simulink model "BALANCEAMENTO_MEDIA"  (Simulink 7.5)
settings: Solver=ode45  StartTime=0.0  StopTime=40000  RelTol=1e-2
libraries: powerlib x49, simulink x1
settings Model: Creator=André  LastModifiedBy=André
settings SolverCC: ZeroCrossAlgorithm=Adaptive

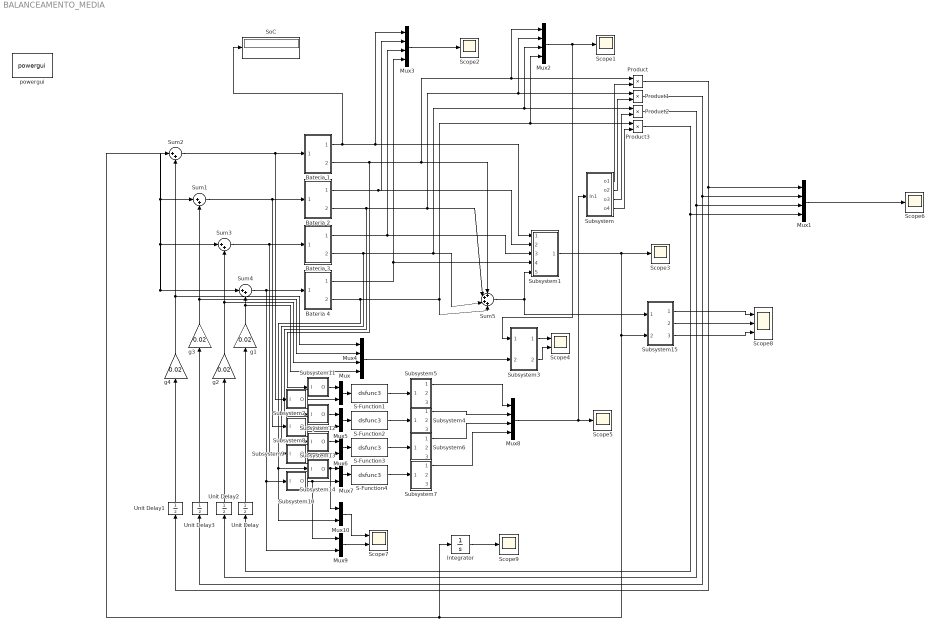
== system BALANCEAMENTO_MEDIA ==
  Bateria 1 : Subsystem
  Bateria 2 : Subsystem
  Bateria 3 : Subsystem
  Bateria 4 : Subsystem
  Integrator : Integrator
  Mux{,5..7,9..10} (6 alike) : Mux  Inputs=2
  Mux{1..4,8} (5 alike) : Mux
  Product{,1..3} (4 alike) : Product  OutDataType=fixdt(1, 16)  OutScaling=2^0  RndMeth=Zero
  S-Function{1..4} (4 alike) : S-Function  FunctionName=dsfunc3  Parameters="[0.5  0.01 0.01 1] %1 para UKF, 2 para EKF"  EnableBusSupport=off
  Scope{1..3,5..6,9} (6 alike) : Scope
      Scope1 settings: TimeRange=3600  YMin=3.34  YMax=3.361  SaveName=Volt
      Scope2 settings: TimeRange=1000  YMin=0.375  YMax=0.925  SaveName=SoC
      Scope3 settings: TimeRange=3600  YMin=0.40252  YMax=0.40262  SaveName=corrente
      Scope5 settings: TimeRange=1000  YMin=0.5  YMax=0.825  SaveName=SoC1
      Scope6 settings: TimeRange=3600  YMin=0  YMax=3.25  SaveName=ScopeData7
      Scope9 settings: TimeRange=1000  YMin=219  YMax=232  SaveName=CAP
  Scope4 : Scope  NumInputPorts=2
      settings: TimeRange=3600  YMin=0~7074.25  YMax=0.25~7076.75  SaveName=energia
  Scope7 : Scope  NumInputPorts=2
      settings: TimeRange=1000  YMin=3.025~0.325  YMax=3.225~0.5  SaveName=CV
  Scope8 : Scope  NumInputPorts=3
      settings: TimeRange=3600  YMin=-0.025~3350~-5  YMax=0.25~3800~5  SaveName=energia1
  SoC : Display
  Subsystem : Subsystem
  Subsystem1 : Subsystem
  Subsystem10 : Subsystem
  Subsystem11 : Subsystem
  Subsystem12 : Subsystem
  Subsystem13 : Subsystem
  Subsystem14 : Subsystem
  Subsystem15 : Subsystem
  Subsystem2 : Subsystem
  Subsystem3 : Subsystem
  Subsystem4 : Subsystem
  Subsystem5 : Subsystem
  Subsystem6 : Subsystem
  Subsystem7 : Subsystem
  Subsystem8 : Subsystem
  Subsystem9 : Subsystem
  Sum{1..4} (4 alike) : Sum  Inputs=|++  OutDataType=fixdt(1, 16)  OutScaling=2^0
  Sum5 : Sum  Inputs=++++  OutDataType=fixdt(1, 16)  OutScaling=2^0
  Unit Delay{,1..3} (4 alike) : UnitDelay  SampleTime=-1
  g{1..4} (4 alike) : Gain  Gain=0.02  ParameterDataType=fixdt(1, 16)  ParameterScaling=2^0  OutDataType=fixdt(1, 16)  OutScaling=2^0
  powergui : powerlib/powergui  Priority=1  SystemSampleTime=-1  SimulationMode=Continuous  SampleTime=50e-6  frequency=60  SPID=off  DisableSnubberDevices=off  DisableRonSwitches=off  DisableVfSwitches=off  SwTol=0  Interpol=off  frequencyindice=0  echomessages=off  HookPort=off  DisplayEquations=off  FunctionMessages=off  EnableUseOfTLC=off  x0status=blocks  RestoreLinks=warning  ResistiveCurrentMeasurement=off  Frange=[0:2:500]  Ylog=off  Xlog=on  ShowGrid=off  save=off  variable=ZData  ZoomFFT=on  StartTime=0.0  cycles=1  DisplayStyle=1  fundamental=60  FreqAxis=off  MaxFrequency=1000  frequencyindicesteady=1  RmsSteady=1  display=off  Ts=0  methode=off
  wires:
  Bateria 1/1(x _1) -> SoC/1, Mux3/1, Subsystem1/1(In1)
  Bateria 3/1(x _1) -> Mux3/3, Subsystem1/3(In3)
  Bateria 4/1(x _1) -> Mux3/4, Subsystem1/4(In4)
  Sum1/1 -> Bateria 2/1(u_1), Subsystem8/1(I)
  Subsystem/1(o1) -> Product/2
  Sum2/1 -> Bateria 1/1(u_1), Subsystem2/1(I)
  Subsystem/2(o2) -> Product1/2
  Sum3/1 -> Bateria 3/1(u_1), Subsystem9/1(I)
  Subsystem/3(o3) -> Product2/2
  Sum4/1 -> Bateria 4/1(u_1), Subsystem10/1(I), Mux9/2
  Subsystem/4(o4) -> Product3/2
  Bateria 1/2(y _1) -> Mux2/1, Product/1, Sum5/1, Subsystem11/1(I)
  Bateria 2/2(y _1) -> Product1/1, Mux2/2, Sum5/2, Subsystem12/1(I)
  Bateria 3/2(y _1) -> Product2/1, Mux2/3, Sum5/3, Subsystem13/1(I)
  Bateria 4/2(y _1) -> Product3/1, Mux2/4, Sum5/4, Subsystem14/1(I), Mux10/2
  Bateria 2/1(x _1) -> Mux3/2, Subsystem1/2(In2)
  Product3/1 -> Mux1/4, Unit Delay/1
  Product2/1 -> Mux1/3, Unit Delay2/1
  Product1/1 -> Mux1/2, Unit Delay3/1
  Product/1 -> Mux1/1, Unit Delay1/1
  g1/1 -> Sum4/2, Mux4/4
  g2/1 -> Sum3/2, Mux4/3
  g3/1 -> Sum1/2, Mux4/2
  g4/1 -> Sum2/2, Mux4/1
  Mux2/1 -> Scope1/1, Subsystem3/1(In1)
  Mux3/1 -> Scope2/1
  Sum5/1 -> Subsystem1/5(In5), Subsystem15/1(In1)
  Subsystem1/1(Corrente) -> Scope3/1, Subsystem15/2(In2), Sum2/1, Sum3/1, Sum4/1, Sum1/1, Integrator/1
  Mux1/1 -> Scope6/1
  Subsystem3/1(Pot) -> Scope4/1
  Subsystem3/2(Energ) -> Scope4/2
  Mux4/1 -> Subsystem3/2(In2)
  S-Function1/1 -> Subsystem5/1(1)
  Mux/1 -> S-Function1/1
  S-Function2/1 -> Subsystem4/1(1)
  Mux5/1 -> S-Function2/1
  S-Function3/1 -> Subsystem6/1(1)
  Mux6/1 -> S-Function3/1
  S-Function4/1 -> Subsystem7/1(1)
  Mux7/1 -> S-Function4/1
  Mux8/1 -> Scope5/1, Subsystem/1(In1)
  Subsystem5/1(1-) -> Mux8/1
  Subsystem4/1(1-) -> Mux8/2
  Subsystem6/1(1-) -> Mux8/3
  Subsystem7/1(1-) -> Mux8/4
  Unit Delay1/1 -> g4/1
  Unit Delay3/1 -> g3/1
  Unit Delay2/1 -> g2/1
  Unit Delay/1 -> g1/1
  Subsystem2/1(O) -> Mux/2
  Subsystem8/1(O) -> Mux5/2
  Subsystem9/1(O) -> Mux6/2
  Subsystem10/1(O) -> Mux7/2, Mux9/1
  Subsystem11/1(O) -> Mux/1
  Subsystem12/1(O) -> Mux5/1
  Subsystem13/1(O) -> Mux6/1
  Subsystem14/1(O) -> Mux7/1, Mux10/1
  Mux9/1 -> Scope7/2
  Mux10/1 -> Scope7/1
  Subsystem15/1(Pot) -> Scope8/1
  Subsystem15/2(Energ) -> Scope8/2
  Subsystem15/3(Energ1) -> Scope8/3
  Integrator/1 -> Scope9/1

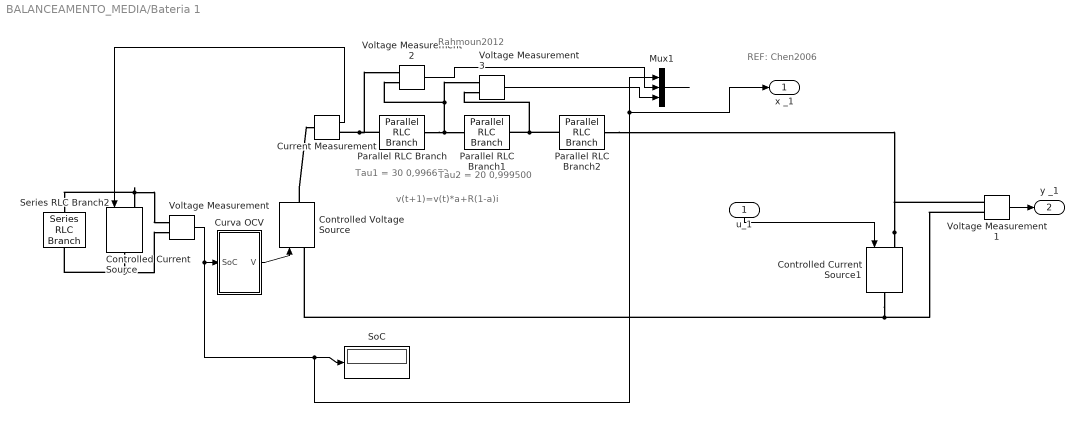
== system BALANCEAMENTO_MEDIA/Bateria 1 ==
  note: REF: Chen2006
  note: Tau1 = 30
      | 0,996672
  note: Tau2 = 20
      | 0,999500
  note: Rahmoun2012
  note: v(t+1)=v(t)*a+R(1-a)i
  u_1 : Inport
  Controlled Current Source : powerlib/Electrical Sources/Controlled Current Source  DialogController=POWERSYS.PowerSysDialog  SystemSampleTime=-1  Initialize=on  Source_Type=AC  Amplitude=0  Phase=0  Frequency=0  Measurements=None
  Controlled Current Source1 : powerlib/Electrical Sources/Controlled Current Source  DialogController=POWERSYS.PowerSysDialog  SystemSampleTime=-1  Initialize=on  Source_Type=DC  Amplitude=0  Phase=0  Frequency=0  Measurements=None
  Controlled Voltage Source : powerlib/Electrical Sources/Controlled Voltage Source  DialogController=POWERSYS.PowerSysDialog  SystemSampleTime=-1  Initialize=on  Source_Type=AC  Amplitude=0  Phase=0  Frequency=0  Measurements=None
  Current Measurement : powerlib/Measurements/Current Measurement  DialogController=POWERSYS.PowerSysDialog  SystemSampleTime=-1  PhasorSimulation=off  OutputType=Complex  PSBequivalent=0
  Curva OCV : Subsystem
  Mux1 : Mux  Inputs=3
  Parallel RLC Branch : powerlib/Elements/Parallel RLC Branch  DialogController=POWERSYS.PowerSysDialog  PhysicalDomain=powersysdomain  SubClassName=unknown  LeftPortType=p1  RightPortType=p1  LConnTagsString=a  RConnTagsString=__new0  BranchType=RC  Resistance=0.115  Inductance=1e-3  SetiL0=off  InitialCurrent=0  Capacitance=600  Setx0=off  InitialVoltage=0  Measurements=None
  Parallel RLC Branch1 : powerlib/Elements/Parallel RLC Branch  DialogController=POWERSYS.PowerSysDialog  PhysicalDomain=powersysdomain  SubClassName=unknown  LeftPortType=p1  RightPortType=p1  LConnTagsString=a  RConnTagsString=__new0  BranchType=RC  Resistance=0.066  Inductance=1e-3  SetiL0=off  InitialCurrent=0  Capacitance=409.1  Setx0=off  InitialVoltage=0  Measurements=None
  Parallel RLC Branch2 : powerlib/Elements/Parallel RLC Branch  DialogController=POWERSYS.PowerSysDialog  PhysicalDomain=powersysdomain  SubClassName=unknown  LeftPortType=p1  RightPortType=p1  LConnTagsString=a  RConnTagsString=__new0  BranchType=R  Resistance=0.174  Inductance=1e-3  SetiL0=off  InitialCurrent=0  Capacitance=1e-6  Setx0=off  InitialVoltage=0  Measurements=None
  Series RLC Branch2 : powerlib/Elements/Series RLC Branch  DialogController=POWERSYS.PowerSysDialog  PhysicalDomain=powersysdomain  SubClassName=unknown  LeftPortType=p1  RightPortType=p1  LConnTagsString=__new0  RConnTagsString=__new0  BranchType=C  Resistance=1  Inductance=1e-3  SetiL0=off  InitialCurrent=0  Capacitance=2070  Setx0=on  InitialVoltage=0.98  Measurements=None
  SoC : Display
  Voltage Measurement{,1..3} (4 alike) : powerlib/Measurements/Voltage Measurement  DialogController=POWERSYS.PowerSysDialog  SystemSampleTime=-1  PhasorSimulation=off  OutputType=Complex  PSBequivalent=0
  x _1 : Outport
  y _1 : Outport  Port=2
  wires:
  Voltage Measurement1/1 -> y _1/1
  Curva OCV/1(V) -> Controlled Voltage Source/1
  Voltage Measurement/1 -> Curva OCV/1(SoC), SoC/1, Mux1/1, x _1/1
  Current Measurement/1 -> Controlled Current Source/1
  u_1/1 -> Controlled Current Source1/1
  Mux1/1 -> ?
  Voltage Measurement2/1 -> Mux1/2
  Voltage Measurement3/1 -> Mux1/3
  connections:
  Controlled Current Source/LConn1 -- Voltage Measurement/LConn1 -- Series RLC Branch2/LConn1
  Controlled Current Source/RConn1 -- Voltage Measurement/LConn2 -- Series RLC Branch2/RConn1
  Controlled Current Source1/LConn1 -- Parallel RLC Branch2/RConn1 -- Voltage Measurement1/LConn1
  Controlled Current Source1/RConn1 -- Controlled Voltage Source/LConn1 -- Voltage Measurement1/LConn2
  Controlled Voltage Source/RConn1 -- Current Measurement/LConn1
  Parallel RLC Branch/LConn1 -- Current Measurement/RConn1 -- Voltage Measurement2/LConn1
  Parallel RLC Branch/RConn1 -- Parallel RLC Branch1/LConn1 -- Voltage Measurement2/LConn2 -- Voltage Measurement3/LConn1
  Parallel RLC Branch2/LConn1 -- Parallel RLC Branch1/RConn1 -- Voltage Measurement3/LConn2

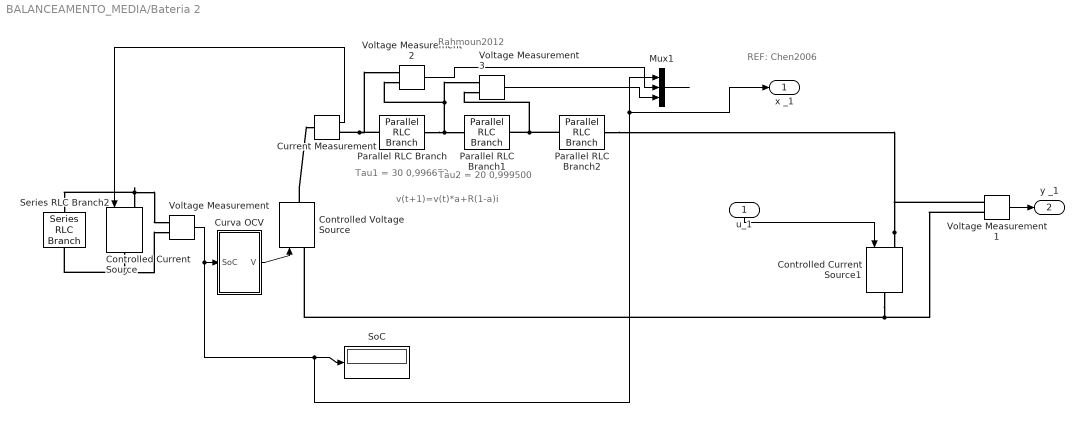
== system BALANCEAMENTO_MEDIA/Bateria 2 ==
  note: REF: Chen2006
  note: Tau1 = 30
      | 0,996672
  note: Tau2 = 20
      | 0,999500
  note: Rahmoun2012
  note: v(t+1)=v(t)*a+R(1-a)i
  u_1 : Inport
  Controlled Current Source : powerlib/Electrical Sources/Controlled Current Source  DialogController=POWERSYS.PowerSysDialog  SystemSampleTime=-1  Initialize=on  Source_Type=AC  Amplitude=0  Phase=0  Frequency=0  Measurements=None
  Controlled Current Source1 : powerlib/Electrical Sources/Controlled Current Source  DialogController=POWERSYS.PowerSysDialog  SystemSampleTime=-1  Initialize=on  Source_Type=DC  Amplitude=0  Phase=0  Frequency=0  Measurements=None
  Controlled Voltage Source : powerlib/Electrical Sources/Controlled Voltage Source  DialogController=POWERSYS.PowerSysDialog  SystemSampleTime=-1  Initialize=on  Source_Type=AC  Amplitude=0  Phase=0  Frequency=0  Measurements=None
  Current Measurement : powerlib/Measurements/Current Measurement  DialogController=POWERSYS.PowerSysDialog  SystemSampleTime=-1  PhasorSimulation=off  OutputType=Complex  PSBequivalent=0
  Curva OCV : Subsystem
  Mux1 : Mux  Inputs=3
  Parallel RLC Branch : powerlib/Elements/Parallel RLC Branch  DialogController=POWERSYS.PowerSysDialog  PhysicalDomain=powersysdomain  SubClassName=unknown  LeftPortType=p1  RightPortType=p1  LConnTagsString=a  RConnTagsString=__new0  BranchType=RC  Resistance=0.115  Inductance=1e-3  SetiL0=off  InitialCurrent=0  Capacitance=600  Setx0=off  InitialVoltage=0  Measurements=None
  Parallel RLC Branch1 : powerlib/Elements/Parallel RLC Branch  DialogController=POWERSYS.PowerSysDialog  PhysicalDomain=powersysdomain  SubClassName=unknown  LeftPortType=p1  RightPortType=p1  LConnTagsString=a  RConnTagsString=__new0  BranchType=RC  Resistance=0.066  Inductance=1e-3  SetiL0=off  InitialCurrent=0  Capacitance=409.1  Setx0=off  InitialVoltage=0  Measurements=None
  Parallel RLC Branch2 : powerlib/Elements/Parallel RLC Branch  DialogController=POWERSYS.PowerSysDialog  PhysicalDomain=powersysdomain  SubClassName=unknown  LeftPortType=p1  RightPortType=p1  LConnTagsString=a  RConnTagsString=__new0  BranchType=R  Resistance=0.174  Inductance=1e-3  SetiL0=off  InitialCurrent=0  Capacitance=1e-6  Setx0=off  InitialVoltage=0  Measurements=None
  Series RLC Branch2 : powerlib/Elements/Series RLC Branch  DialogController=POWERSYS.PowerSysDialog  PhysicalDomain=powersysdomain  SubClassName=unknown  LeftPortType=p1  RightPortType=p1  LConnTagsString=__new0  RConnTagsString=__new0  BranchType=C  Resistance=1  Inductance=1e-3  SetiL0=off  InitialCurrent=0  Capacitance=2070*0.9  Setx0=on  InitialVoltage=0.90  Measurements=None
  SoC : Display
  Voltage Measurement{,1..3} (4 alike) : powerlib/Measurements/Voltage Measurement  DialogController=POWERSYS.PowerSysDialog  SystemSampleTime=-1  PhasorSimulation=off  OutputType=Complex  PSBequivalent=0
  x _1 : Outport
  y _1 : Outport  Port=2
  wires:
  Voltage Measurement1/1 -> y _1/1
  Curva OCV/1(V) -> Controlled Voltage Source/1
  Voltage Measurement/1 -> Curva OCV/1(SoC), SoC/1, Mux1/1, x _1/1
  Current Measurement/1 -> Controlled Current Source/1
  u_1/1 -> Controlled Current Source1/1
  Mux1/1 -> ?
  Voltage Measurement2/1 -> Mux1/2
  Voltage Measurement3/1 -> Mux1/3
  connections:
  Controlled Current Source/LConn1 -- Voltage Measurement/LConn1 -- Series RLC Branch2/LConn1
  Controlled Current Source/RConn1 -- Voltage Measurement/LConn2 -- Series RLC Branch2/RConn1
  Controlled Current Source1/LConn1 -- Parallel RLC Branch2/RConn1 -- Voltage Measurement1/LConn1
  Controlled Current Source1/RConn1 -- Controlled Voltage Source/LConn1 -- Voltage Measurement1/LConn2
  Controlled Voltage Source/RConn1 -- Current Measurement/LConn1
  Parallel RLC Branch/LConn1 -- Current Measurement/RConn1 -- Voltage Measurement2/LConn1
  Parallel RLC Branch/RConn1 -- Parallel RLC Branch1/LConn1 -- Voltage Measurement2/LConn2 -- Voltage Measurement3/LConn1
  Parallel RLC Branch2/LConn1 -- Parallel RLC Branch1/RConn1 -- Voltage Measurement3/LConn2

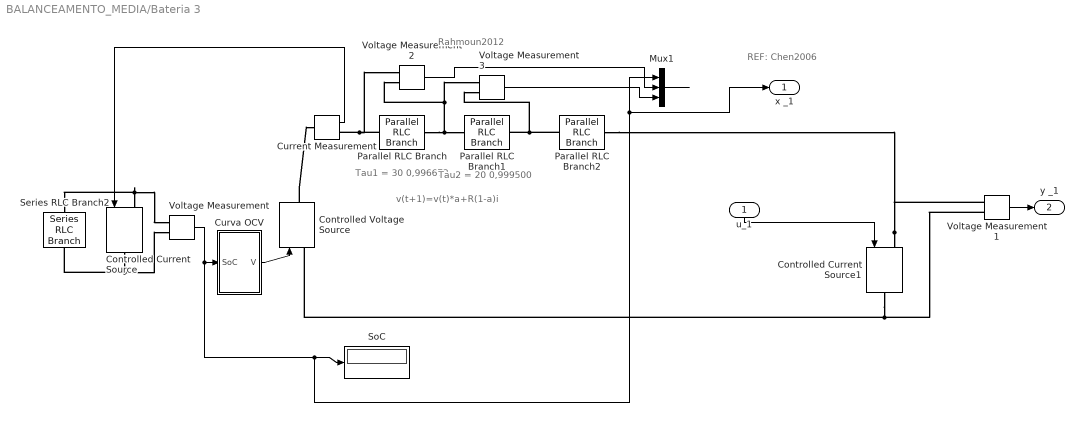
== system BALANCEAMENTO_MEDIA/Bateria 3 ==
  note: REF: Chen2006
  note: Tau1 = 30
      | 0,996672
  note: Tau2 = 20
      | 0,999500
  note: Rahmoun2012
  note: v(t+1)=v(t)*a+R(1-a)i
  u_1 : Inport
  Controlled Current Source : powerlib/Electrical Sources/Controlled Current Source  DialogController=POWERSYS.PowerSysDialog  SystemSampleTime=-1  Initialize=on  Source_Type=AC  Amplitude=0  Phase=0  Frequency=0  Measurements=None
  Controlled Current Source1 : powerlib/Electrical Sources/Controlled Current Source  DialogController=POWERSYS.PowerSysDialog  SystemSampleTime=-1  Initialize=on  Source_Type=DC  Amplitude=0  Phase=0  Frequency=0  Measurements=None
  Controlled Voltage Source : powerlib/Electrical Sources/Controlled Voltage Source  DialogController=POWERSYS.PowerSysDialog  SystemSampleTime=-1  Initialize=on  Source_Type=AC  Amplitude=0  Phase=0  Frequency=0  Measurements=None
  Current Measurement : powerlib/Measurements/Current Measurement  DialogController=POWERSYS.PowerSysDialog  SystemSampleTime=-1  PhasorSimulation=off  OutputType=Complex  PSBequivalent=0
  Curva OCV : Subsystem
  Mux1 : Mux  Inputs=3
  Parallel RLC Branch : powerlib/Elements/Parallel RLC Branch  DialogController=POWERSYS.PowerSysDialog  PhysicalDomain=powersysdomain  SubClassName=unknown  LeftPortType=p1  RightPortType=p1  LConnTagsString=a  RConnTagsString=__new0  BranchType=RC  Resistance=0.115  Inductance=1e-3  SetiL0=off  InitialCurrent=0  Capacitance=600  Setx0=off  InitialVoltage=0  Measurements=None
  Parallel RLC Branch1 : powerlib/Elements/Parallel RLC Branch  DialogController=POWERSYS.PowerSysDialog  PhysicalDomain=powersysdomain  SubClassName=unknown  LeftPortType=p1  RightPortType=p1  LConnTagsString=a  RConnTagsString=__new0  BranchType=RC  Resistance=0.066  Inductance=1e-3  SetiL0=off  InitialCurrent=0  Capacitance=409.1  Setx0=off  InitialVoltage=0  Measurements=None
  Parallel RLC Branch2 : powerlib/Elements/Parallel RLC Branch  DialogController=POWERSYS.PowerSysDialog  PhysicalDomain=powersysdomain  SubClassName=unknown  LeftPortType=p1  RightPortType=p1  LConnTagsString=a  RConnTagsString=__new0  BranchType=R  Resistance=0.174  Inductance=1e-3  SetiL0=off  InitialCurrent=0  Capacitance=1e-6  Setx0=off  InitialVoltage=0  Measurements=None
  Series RLC Branch2 : powerlib/Elements/Series RLC Branch  DialogController=POWERSYS.PowerSysDialog  PhysicalDomain=powersysdomain  SubClassName=unknown  LeftPortType=p1  RightPortType=p1  LConnTagsString=__new0  RConnTagsString=__new0  BranchType=C  Resistance=1  Inductance=1e-3  SetiL0=off  InitialCurrent=0  Capacitance=2070  Setx0=on  InitialVoltage=0.80  Measurements=None
  SoC : Display
  Voltage Measurement{,1..3} (4 alike) : powerlib/Measurements/Voltage Measurement  DialogController=POWERSYS.PowerSysDialog  SystemSampleTime=-1  PhasorSimulation=off  OutputType=Complex  PSBequivalent=0
  x _1 : Outport
  y _1 : Outport  Port=2
  wires:
  Voltage Measurement1/1 -> y _1/1
  Curva OCV/1(V) -> Controlled Voltage Source/1
  Voltage Measurement/1 -> Curva OCV/1(SoC), SoC/1, Mux1/1, x _1/1
  Current Measurement/1 -> Controlled Current Source/1
  u_1/1 -> Controlled Current Source1/1
  Mux1/1 -> ?
  Voltage Measurement2/1 -> Mux1/2
  Voltage Measurement3/1 -> Mux1/3
  connections:
  Controlled Current Source/LConn1 -- Voltage Measurement/LConn1 -- Series RLC Branch2/LConn1
  Controlled Current Source/RConn1 -- Voltage Measurement/LConn2 -- Series RLC Branch2/RConn1
  Controlled Current Source1/LConn1 -- Parallel RLC Branch2/RConn1 -- Voltage Measurement1/LConn1
  Controlled Current Source1/RConn1 -- Controlled Voltage Source/LConn1 -- Voltage Measurement1/LConn2
  Controlled Voltage Source/RConn1 -- Current Measurement/LConn1
  Parallel RLC Branch/LConn1 -- Current Measurement/RConn1 -- Voltage Measurement2/LConn1
  Parallel RLC Branch/RConn1 -- Parallel RLC Branch1/LConn1 -- Voltage Measurement2/LConn2 -- Voltage Measurement3/LConn1
  Parallel RLC Branch2/LConn1 -- Parallel RLC Branch1/RConn1 -- Voltage Measurement3/LConn2

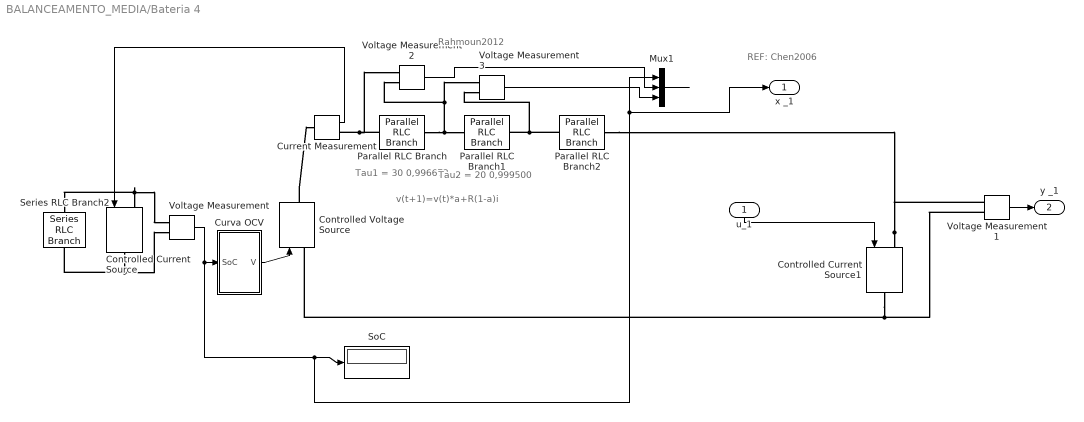
== system BALANCEAMENTO_MEDIA/Bateria 4 ==
  note: REF: Chen2006
  note: Tau1 = 30
      | 0,996672
  note: Tau2 = 20
      | 0,999500
  note: Rahmoun2012
  note: v(t+1)=v(t)*a+R(1-a)i
  u_1 : Inport
  Controlled Current Source : powerlib/Electrical Sources/Controlled Current Source  DialogController=POWERSYS.PowerSysDialog  SystemSampleTime=-1  Initialize=on  Source_Type=AC  Amplitude=0  Phase=0  Frequency=0  Measurements=None
  Controlled Current Source1 : powerlib/Electrical Sources/Controlled Current Source  DialogController=POWERSYS.PowerSysDialog  SystemSampleTime=-1  Initialize=on  Source_Type=DC  Amplitude=0  Phase=0  Frequency=0  Measurements=None
  Controlled Voltage Source : powerlib/Electrical Sources/Controlled Voltage Source  DialogController=POWERSYS.PowerSysDialog  SystemSampleTime=-1  Initialize=on  Source_Type=AC  Amplitude=0  Phase=0  Frequency=0  Measurements=None
  Current Measurement : powerlib/Measurements/Current Measurement  DialogController=POWERSYS.PowerSysDialog  SystemSampleTime=-1  PhasorSimulation=off  OutputType=Complex  PSBequivalent=0
  Curva OCV : Subsystem
  Mux1 : Mux  Inputs=3
  Parallel RLC Branch : powerlib/Elements/Parallel RLC Branch  DialogController=POWERSYS.PowerSysDialog  PhysicalDomain=powersysdomain  SubClassName=unknown  LeftPortType=p1  RightPortType=p1  LConnTagsString=a  RConnTagsString=__new0  BranchType=RC  Resistance=0.115  Inductance=1e-3  SetiL0=off  InitialCurrent=0  Capacitance=600  Setx0=off  InitialVoltage=0  Measurements=None
  Parallel RLC Branch1 : powerlib/Elements/Parallel RLC Branch  DialogController=POWERSYS.PowerSysDialog  PhysicalDomain=powersysdomain  SubClassName=unknown  LeftPortType=p1  RightPortType=p1  LConnTagsString=a  RConnTagsString=__new0  BranchType=RC  Resistance=0.066  Inductance=1e-3  SetiL0=off  InitialCurrent=0  Capacitance=409.1  Setx0=off  InitialVoltage=0  Measurements=None
  Parallel RLC Branch2 : powerlib/Elements/Parallel RLC Branch  DialogController=POWERSYS.PowerSysDialog  PhysicalDomain=powersysdomain  SubClassName=unknown  LeftPortType=p1  RightPortType=p1  LConnTagsString=a  RConnTagsString=__new0  BranchType=R  Resistance=0.174  Inductance=1e-3  SetiL0=off  InitialCurrent=0  Capacitance=1e-6  Setx0=off  InitialVoltage=0  Measurements=None
  Series RLC Branch2 : powerlib/Elements/Series RLC Branch  DialogController=POWERSYS.PowerSysDialog  PhysicalDomain=powersysdomain  SubClassName=unknown  LeftPortType=p1  RightPortType=p1  LConnTagsString=__new0  RConnTagsString=__new0  BranchType=C  Resistance=1  Inductance=1e-3  SetiL0=off  InitialCurrent=0  Capacitance=2070  Setx0=on  InitialVoltage=0.70  Measurements=None
  SoC : Display
  Voltage Measurement{,1..3} (4 alike) : powerlib/Measurements/Voltage Measurement  DialogController=POWERSYS.PowerSysDialog  SystemSampleTime=-1  PhasorSimulation=off  OutputType=Complex  PSBequivalent=0
  x _1 : Outport
  y _1 : Outport  Port=2
  wires:
  Voltage Measurement1/1 -> y _1/1
  Curva OCV/1(V) -> Controlled Voltage Source/1
  Voltage Measurement/1 -> Curva OCV/1(SoC), SoC/1, Mux1/1, x _1/1
  Current Measurement/1 -> Controlled Current Source/1
  u_1/1 -> Controlled Current Source1/1
  Mux1/1 -> ?
  Voltage Measurement2/1 -> Mux1/2
  Voltage Measurement3/1 -> Mux1/3
  connections:
  Controlled Current Source/LConn1 -- Voltage Measurement/LConn1 -- Series RLC Branch2/LConn1
  Controlled Current Source/RConn1 -- Voltage Measurement/LConn2 -- Series RLC Branch2/RConn1
  Controlled Current Source1/LConn1 -- Parallel RLC Branch2/RConn1 -- Voltage Measurement1/LConn1
  Controlled Current Source1/RConn1 -- Controlled Voltage Source/LConn1 -- Voltage Measurement1/LConn2
  Controlled Voltage Source/RConn1 -- Current Measurement/LConn1
  Parallel RLC Branch/LConn1 -- Current Measurement/RConn1 -- Voltage Measurement2/LConn1
  Parallel RLC Branch/RConn1 -- Parallel RLC Branch1/LConn1 -- Voltage Measurement2/LConn2 -- Voltage Measurement3/LConn1
  Parallel RLC Branch2/LConn1 -- Parallel RLC Branch1/RConn1 -- Voltage Measurement3/LConn2

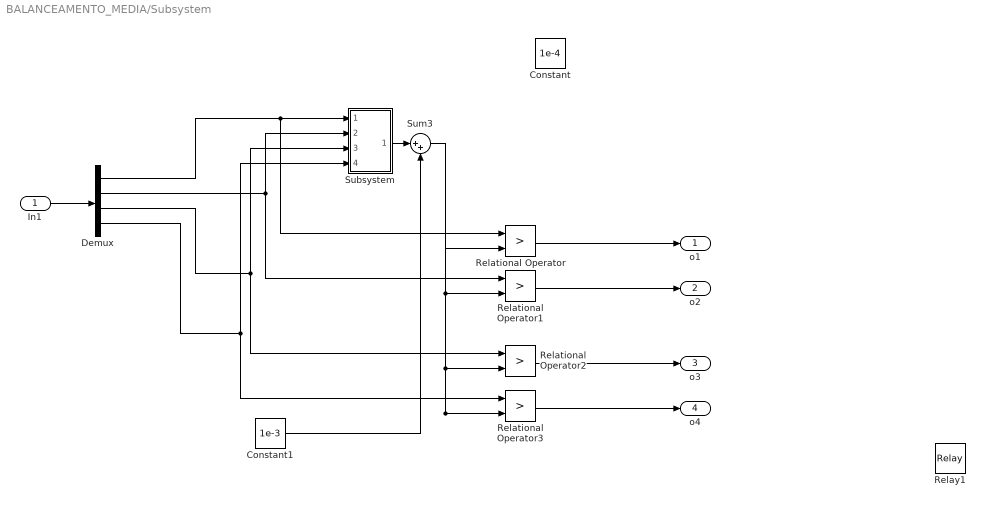
== system BALANCEAMENTO_MEDIA/Subsystem ==
  In1 : Inport
  Constant : Constant  Value=1e-4  OutDataType=fixdt(1, 16)  OutScaling=2^0
  Constant1 : Constant  Value=1e-3  OutDataType=fixdt(1, 16)  OutScaling=2^0
  Demux : Demux
  Relational Operator{,1..3} (4 alike) : RelationalOperator  Operator=>  LogicOutDataTypeMode=boolean  LogicDataType=fixdt(0, 8)  OutDataTypeStr=boolean
  Relay1 : Relay  OnSwitchValue=1e-8  OffSwitchValue=0  OnOutputValue=-1  OutDataType=fixdt(1, 16)  OutScaling=2^0
  Subsystem : Subsystem
  Sum3 : Sum  Inputs=|++  OutDataType=fixdt(1, 16)  OutScaling=2^0
  o1 : Outport
  o2 : Outport  Port=2
  o3 : Outport  Port=3
  o4 : Outport  Port=4
  wires:
  Demux/1 -> Relational Operator/1, Subsystem/1(In1)
  Demux/2 -> Relational Operator1/1, Subsystem/2(In2)
  Demux/3 -> Relational Operator2/1, Subsystem/3(In3)
  Demux/4 -> Relational Operator3/1, Subsystem/4(In4)
  Sum3/1 -> Relational Operator/2, Relational Operator1/2, Relational Operator2/2, Relational Operator3/2
  Relational Operator/1 -> o1/1
  Relational Operator1/1 -> o2/1
  Relational Operator2/1 -> o3/1
  Relational Operator3/1 -> o4/1
  Subsystem/1(Out1) -> Sum3/1
  Constant1/1 -> Sum3/2
  In1/1 -> Demux/1

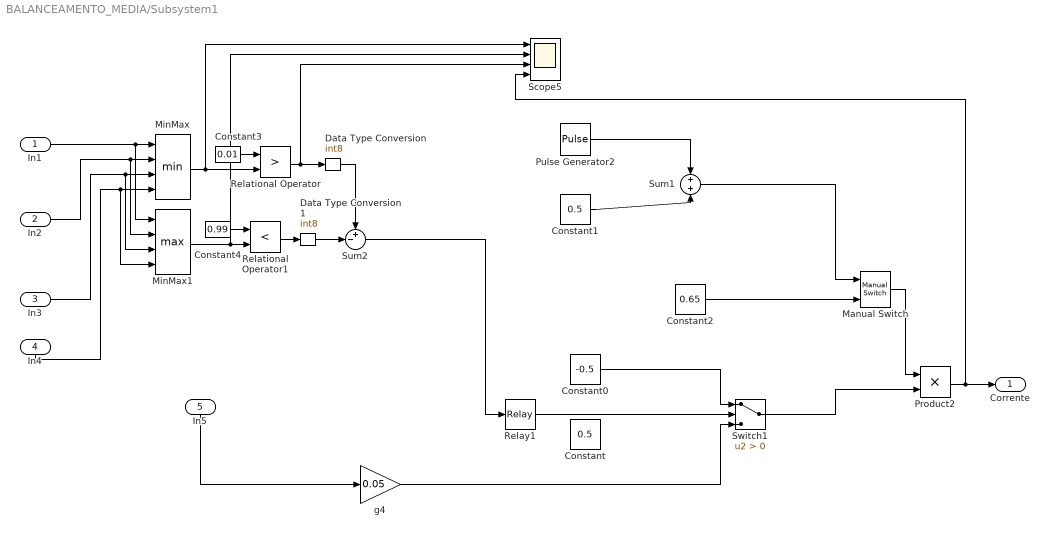
== system BALANCEAMENTO_MEDIA/Subsystem1 ==
  In1 : Inport
  In2 : Inport  Port=2
  In3 : Inport  Port=3
  In4 : Inport  Port=4
  In5 : Inport  Port=5
  Constant : Constant  Value=0.5  OutDataType=fixdt(1, 16)  OutScaling=2^0
  Constant0 : Constant  Value=-0.5  OutDataType=fixdt(1, 16)  OutScaling=2^0
  Constant1 : Constant  Value=0.5  OutDataType=fixdt(1, 16)  OutScaling=2^0
  Constant2 : Constant  Value=0.65  OutDataType=fixdt(1, 16)  OutScaling=2^0
  Constant3 : Constant  Value=0.01  OutDataType=fixdt(1, 16)  OutScaling=2^0
  Constant4 : Constant  Value=0.99  OutDataType=fixdt(1, 16)  OutScaling=2^0
  Data Type Conversion : DataTypeConversion  OutDataTypeMode=int8  OutDataType=fixdt(1, 16)  OutScaling=2^0  OutDataTypeStr=int8
  Data Type Conversion1 : DataTypeConversion  OutDataTypeMode=int8  OutDataType=fixdt(1, 16)  OutScaling=2^0  OutDataTypeStr=int8
  Manual Switch : simulink/Signal Routing/Manual Switch  SystemSampleTime=-1  sw=0  action=0  varsize=off
  MinMax : MinMax  Inputs=4  OutDataType=fixdt(1, 16)  OutScaling=2^0
  MinMax1 : MinMax  Function=max  Inputs=4  OutDataType=fixdt(1, 16)  OutScaling=2^0
  Product2 : Product  OutDataType=fixdt(1, 16)  OutScaling=2^0  RndMeth=Zero
  Pulse Generator2 : DiscretePulseGenerator  PulseType=Time based  Amplitude=2.3  Period=100  PulseWidth=50  PhaseDelay=0  SampleTime=1
  Relational Operator : RelationalOperator  Operator=>  LogicOutDataTypeMode=boolean  LogicDataType=fixdt(0, 8)  OutDataTypeStr=boolean
  Relational Operator1 : RelationalOperator  Operator=<  LogicOutDataTypeMode=boolean  LogicDataType=fixdt(0, 8)  OutDataTypeStr=boolean
  Relay1 : Relay  OnSwitchValue=0.9  OffSwitchValue=-0.9  OutDataType=fixdt(1, 16)  OutScaling=2^0  ZeroCross=off
  Scope5 : Scope  NumInputPorts=4
      settings: TimeRange=3600  YMin=-3.46945e-018~0.22~0~-0.4  YMax=0.1~0.29~1~0.4  SaveName=ScopeData4
  Sum1 : Sum  OutDataType=fixdt(1, 16)  OutScaling=2^0
  Sum2 : Sum  Inputs=+-|  OutDataType=fixdt(1, 16)  OutScaling=2^0
  Switch1 : Switch  Criteria=u2 > Threshold  OutDataType=fixdt(1, 16)  OutScaling=2^0
  g4 : Gain  Gain=0.05  ParameterDataType=fixdt(1, 16)  ParameterScaling=2^0  OutDataType=fixdt(1, 16)  OutScaling=2^0
  Corrente : Outport
  wires:
  In1/1 -> MinMax/1, MinMax1/1
  In2/1 -> MinMax/2, MinMax1/2
  In3/1 -> MinMax/3, MinMax1/3
  In4/1 -> MinMax/4, MinMax1/4
  Product2/1 -> Corrente/1, Scope5/4
  Pulse Generator2/1 -> Sum1/1
  Sum1/1 -> Manual Switch/1
  Constant1/1 -> Sum1/2
  Manual Switch/1 -> Product2/1
  Relay1/1 -> Switch1/2
  Constant0/1 -> Switch1/1
  Switch1/1 -> Product2/2
  MinMax1/1 -> Relational Operator1/2, Scope5/2
  MinMax/1 -> Relational Operator/2, Scope5/1
  Constant3/1 -> Relational Operator/1
  Constant2/1 -> Manual Switch/2
  In5/1 -> g4/1
  g4/1 -> Switch1/3
  Constant4/1 -> Relational Operator1/1
  Relational Operator/1 -> Data Type Conversion/1, Scope5/3
  Sum2/1 -> Relay1/1
  Data Type Conversion/1 -> Sum2/1
  Relational Operator1/1 -> Data Type Conversion1/1
  Data Type Conversion1/1 -> Sum2/2

== system BALANCEAMENTO_MEDIA/Subsystem10 ==
  I : Inport
  Random Number : RandomNumber  Variance=5e-4  SampleTime=1
  Sum : Sum  Inputs=++|  OutDataType=fixdt(1, 16)  OutScaling=2^0
  O : Outport
  wires:
  Random Number/1 -> Sum/1
  I/1 -> Sum/2
  Sum/1 -> O/1

== system BALANCEAMENTO_MEDIA/Subsystem11 ==
  I : Inport
  Random Number : RandomNumber  Variance=5e-4  SampleTime=1
  Sum : Sum  Inputs=++|  OutDataType=fixdt(1, 16)  OutScaling=2^0
  O : Outport
  wires:
  Random Number/1 -> Sum/1
  I/1 -> Sum/2
  Sum/1 -> O/1

== system BALANCEAMENTO_MEDIA/Subsystem12 ==
  I : Inport
  Random Number : RandomNumber  Variance=5e-4  SampleTime=1
  Sum : Sum  Inputs=++|  OutDataType=fixdt(1, 16)  OutScaling=2^0
  O : Outport
  wires:
  Random Number/1 -> Sum/1
  I/1 -> Sum/2
  Sum/1 -> O/1

== system BALANCEAMENTO_MEDIA/Subsystem13 ==
  I : Inport
  Random Number : RandomNumber  Variance=5e-4  SampleTime=1
  Sum : Sum  Inputs=++|  OutDataType=fixdt(1, 16)  OutScaling=2^0
  O : Outport
  wires:
  Random Number/1 -> Sum/1
  I/1 -> Sum/2
  Sum/1 -> O/1

== system BALANCEAMENTO_MEDIA/Subsystem14 ==
  I : Inport
  Random Number : RandomNumber  Variance=5e-4  SampleTime=1
  Sum : Sum  Inputs=++|  OutDataType=fixdt(1, 16)  OutScaling=2^0
  O : Outport
  wires:
  Random Number/1 -> Sum/1
  I/1 -> Sum/2
  Sum/1 -> O/1

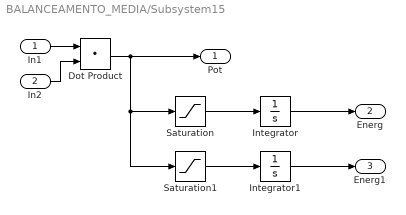
== system BALANCEAMENTO_MEDIA/Subsystem15 ==
  In1 : Inport
  In2 : Inport  Port=2
  Dot Product : DotProduct  OutDataType=fixdt(1, 16)  OutScaling=2^-10  InputSameDT=on  OutDataTypeStr=Inherit: Inherit via internal rule
  Integrator : Integrator
  Integrator1 : Integrator
  Saturation : Saturate  UpperLimit=inf  LowerLimit=0  OutDataType=fixdt(1, 16)  OutScaling=2^0
  Saturation1 : Saturate  UpperLimit=0  LowerLimit=-inf  OutDataType=fixdt(1, 16)  OutScaling=2^0
  Pot : Outport
  Energ : Outport  Port=2
  Energ1 : Outport  Port=3
  wires:
  In1/1 -> Dot Product/1
  In2/1 -> Dot Product/2
  Dot Product/1 -> Pot/1, Saturation/1, Saturation1/1
  Integrator/1 -> Energ/1
  Saturation/1 -> Integrator/1
  Saturation1/1 -> Integrator1/1
  Integrator1/1 -> Energ1/1

== system BALANCEAMENTO_MEDIA/Subsystem2 ==
  I : Inport
  Random Number : RandomNumber  Variance=5e-4  SampleTime=1
  Sum : Sum  Inputs=++|  OutDataType=fixdt(1, 16)  OutScaling=2^0
  O : Outport
  wires:
  Random Number/1 -> Sum/1
  I/1 -> Sum/2
  Sum/1 -> O/1

== system BALANCEAMENTO_MEDIA/Subsystem3 ==
  In1 : Inport
  In2 : Inport  Port=2
  Dot Product : DotProduct  OutDataType=fixdt(1, 16)  OutScaling=2^-10  InputSameDT=on  OutDataTypeStr=Inherit: Inherit via internal rule
  Integrator : Integrator
  Pot : Outport
  Energ : Outport  Port=2
  wires:
  In1/1 -> Dot Product/1
  In2/1 -> Dot Product/2
  Dot Product/1 -> Pot/1, Integrator/1
  Integrator/1 -> Energ/1

== system BALANCEAMENTO_MEDIA/Subsystem4 ==
  1 : Inport
  Demux : Demux  Outputs=7
  Scope3 : Scope  NumInputPorts=3
      settings: TimeRange=10800  YMin=1.38778e-017~8.5e-005~5e-005  YMax=0.225~0.00015~0.0007  SaveName=ScopeData3
  1- : Outport
  2- : Outport  Port=2
  3- : Outport  Port=3
  wires:
  Demux/1 -> 1-/1
  Demux/2 -> 2-/1
  Demux/3 -> 3-/1
  Demux/5 -> Scope3/1
  Demux/6 -> Scope3/2
  Demux/7 -> Scope3/3
  1/1 -> Demux/1

== system BALANCEAMENTO_MEDIA/Subsystem5 ==
  1 : Inport
  Demux : Demux  Outputs=7
  Scope3 : Scope  NumInputPorts=3
      settings: TimeRange=10800  YMin=1.38778e-017~8.5e-005~5e-005  YMax=0.225~0.00015~0.0007  SaveName=ScopeData3
  1- : Outport
  2- : Outport  Port=2
  3- : Outport  Port=3
  wires:
  Demux/1 -> 1-/1
  Demux/2 -> 2-/1
  Demux/3 -> 3-/1
  Demux/5 -> Scope3/1
  Demux/6 -> Scope3/2
  Demux/7 -> Scope3/3
  1/1 -> Demux/1

== system BALANCEAMENTO_MEDIA/Subsystem6 ==
  1 : Inport
  Demux : Demux  Outputs=7
  Scope3 : Scope  NumInputPorts=3
      settings: TimeRange=10800  YMin=1.38778e-017~8.5e-005~5e-005  YMax=0.225~0.00015~0.0007  SaveName=ScopeData3
  1- : Outport
  2- : Outport  Port=2
  3- : Outport  Port=3
  wires:
  Demux/1 -> 1-/1
  Demux/2 -> 2-/1
  Demux/3 -> 3-/1
  Demux/5 -> Scope3/1
  Demux/6 -> Scope3/2
  Demux/7 -> Scope3/3
  1/1 -> Demux/1

== system BALANCEAMENTO_MEDIA/Subsystem7 ==
  1 : Inport
  Demux : Demux  Outputs=7
  Scope3 : Scope  NumInputPorts=3
      settings: TimeRange=10800  YMin=1.38778e-017~8.5e-005~5e-005  YMax=0.225~0.00015~0.0007  SaveName=ScopeData3
  1- : Outport
  2- : Outport  Port=2
  3- : Outport  Port=3
  wires:
  Demux/1 -> 1-/1
  Demux/2 -> 2-/1
  Demux/3 -> 3-/1
  Demux/5 -> Scope3/1
  Demux/6 -> Scope3/2
  Demux/7 -> Scope3/3
  1/1 -> Demux/1

== system BALANCEAMENTO_MEDIA/Subsystem8 ==
  I : Inport
  Random Number : RandomNumber  Variance=5e-4  SampleTime=1
  Sum : Sum  Inputs=++|  OutDataType=fixdt(1, 16)  OutScaling=2^0
  O : Outport
  wires:
  Random Number/1 -> Sum/1
  I/1 -> Sum/2
  Sum/1 -> O/1

== system BALANCEAMENTO_MEDIA/Subsystem9 ==
  I : Inport
  Random Number : RandomNumber  Variance=5e-4  SampleTime=1
  Sum : Sum  Inputs=++|  OutDataType=fixdt(1, 16)  OutScaling=2^0
  O : Outport
  wires:
  Random Number/1 -> Sum/1
  I/1 -> Sum/2
  Sum/1 -> O/1

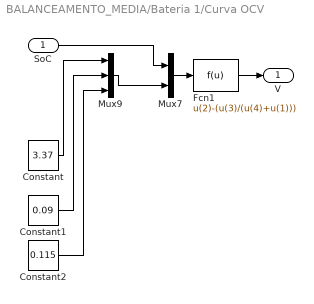
== system BALANCEAMENTO_MEDIA/Bateria 1/Curva OCV ==
  SoC : Inport
  Constant : Constant  Value=3.37  OutDataType=fixdt(1, 16)  OutScaling=2^0
  Constant1 : Constant  Value=0.09  OutDataType=fixdt(1, 16)  OutScaling=2^0
  Constant2 : Constant  Value=0.115  OutDataType=fixdt(1, 16)  OutScaling=2^0
  Fcn1 : Fcn  Expr=u(2)-(u(3)/(u(4)+u(1)))
  Mux7 : Mux  Inputs=2
  Mux9 : Mux  Inputs=3
  V : Outport
  wires:
  Mux9/1 -> Mux7/2
  Constant/1 -> Mux9/1
  Constant1/1 -> Mux9/2
  Constant2/1 -> Mux9/3
  Mux7/1 -> Fcn1/1
  SoC/1 -> Mux7/1
  Fcn1/1 -> V/1

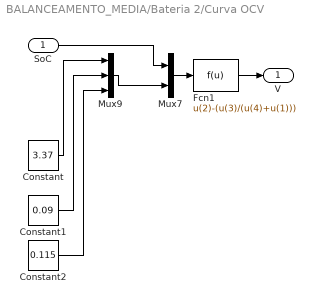
== system BALANCEAMENTO_MEDIA/Bateria 2/Curva OCV ==
  SoC : Inport
  Constant : Constant  Value=3.37  OutDataType=fixdt(1, 16)  OutScaling=2^0
  Constant1 : Constant  Value=0.09  OutDataType=fixdt(1, 16)  OutScaling=2^0
  Constant2 : Constant  Value=0.115  OutDataType=fixdt(1, 16)  OutScaling=2^0
  Fcn1 : Fcn  Expr=u(2)-(u(3)/(u(4)+u(1)))
  Mux7 : Mux  Inputs=2
  Mux9 : Mux  Inputs=3
  V : Outport
  wires:
  Mux9/1 -> Mux7/2
  Constant/1 -> Mux9/1
  Constant1/1 -> Mux9/2
  Constant2/1 -> Mux9/3
  Mux7/1 -> Fcn1/1
  SoC/1 -> Mux7/1
  Fcn1/1 -> V/1

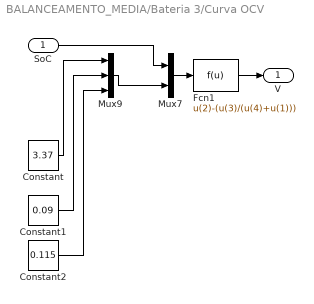
== system BALANCEAMENTO_MEDIA/Bateria 3/Curva OCV ==
  SoC : Inport
  Constant : Constant  Value=3.37  OutDataType=fixdt(1, 16)  OutScaling=2^0
  Constant1 : Constant  Value=0.09  OutDataType=fixdt(1, 16)  OutScaling=2^0
  Constant2 : Constant  Value=0.115  OutDataType=fixdt(1, 16)  OutScaling=2^0
  Fcn1 : Fcn  Expr=u(2)-(u(3)/(u(4)+u(1)))
  Mux7 : Mux  Inputs=2
  Mux9 : Mux  Inputs=3
  V : Outport
  wires:
  Mux9/1 -> Mux7/2
  Constant/1 -> Mux9/1
  Constant1/1 -> Mux9/2
  Constant2/1 -> Mux9/3
  Mux7/1 -> Fcn1/1
  SoC/1 -> Mux7/1
  Fcn1/1 -> V/1

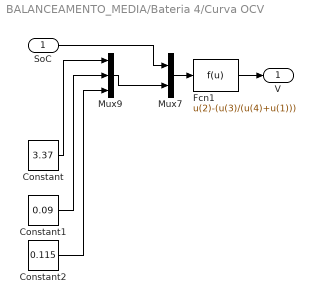
== system BALANCEAMENTO_MEDIA/Bateria 4/Curva OCV ==
  SoC : Inport
  Constant : Constant  Value=3.37  OutDataType=fixdt(1, 16)  OutScaling=2^0
  Constant1 : Constant  Value=0.09  OutDataType=fixdt(1, 16)  OutScaling=2^0
  Constant2 : Constant  Value=0.115  OutDataType=fixdt(1, 16)  OutScaling=2^0
  Fcn1 : Fcn  Expr=u(2)-(u(3)/(u(4)+u(1)))
  Mux7 : Mux  Inputs=2
  Mux9 : Mux  Inputs=3
  V : Outport
  wires:
  Mux9/1 -> Mux7/2
  Constant/1 -> Mux9/1
  Constant1/1 -> Mux9/2
  Constant2/1 -> Mux9/3
  Mux7/1 -> Fcn1/1
  SoC/1 -> Mux7/1
  Fcn1/1 -> V/1

== system BALANCEAMENTO_MEDIA/Subsystem/Subsystem ==
  In1 : Inport
  In2 : Inport  Port=2
  In3 : Inport  Port=3
  In4 : Inport  Port=4
  Sum5 : Sum  Inputs=++++  OutDataType=fixdt(1, 16)  OutScaling=2^0
  g1 : Gain  Gain=1/4  ParameterDataType=fixdt(1, 16)  ParameterScaling=2^0  OutDataType=fixdt(1, 16)  OutScaling=2^0
  Out1 : Outport
  wires:
  Sum5/1 -> g1/1
  In1/1 -> Sum5/1
  In2/1 -> Sum5/2
  g1/1 -> Out1/1
  In3/1 -> Sum5/3
  In4/1 -> Sum5/4
